simulink model "fcn"  (R2019a)
settings: Solver=VariableStepAuto  StartTime=0.0  StopTime=100  RelTol=1e-3
values from neighbouring files (symbols this model uses):
  x0 = [0;0;0;0]    [Script.m]
undefined symbols (not defined in the file or in its folder): params
settings Model: Creator=pc  LastModifiedBy=pc

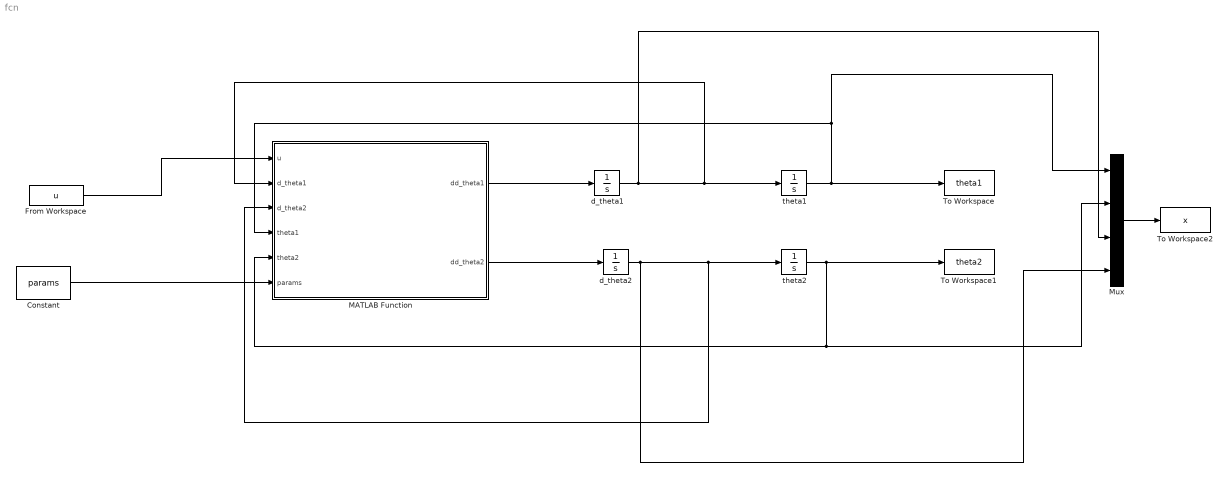
== system fcn ==
  Constant : Constant  Value=params  OutDataTypeStr=Bus: params_bus
  From Workspace : FromWorkspace  VariableName=u  SampleTime=0
  MATLAB Function : MATLAB Function  TreatAsAtomicUnit=on
  Mux : Mux
  To Workspace : ToWorkspace  VariableName=theta1  SaveFormat=Timeseries  SampleTime=-1
  To Workspace1 : ToWorkspace  VariableName=theta2  SaveFormat=Timeseries  SampleTime=-1
  To Workspace2 : ToWorkspace  VariableName=x  SaveFormat=Timeseries  SampleTime=-1
  d_theta1 : Integrator  InitialCondition=x0(2)
  d_theta2 : Integrator  InitialCondition=x0(4)
  theta1 : Integrator  InitialCondition=x0(1)
  theta2 : Integrator  InitialCondition=x0(3)
  wires:
  MATLAB Function/1(dd_theta1) -> d_theta1/1
  MATLAB Function/2(dd_theta2) -> d_theta2/1
  theta2/1 -> Mux/2, MATLAB Function/5(theta2), To Workspace1/1
  Constant/1 -> MATLAB Function/6(params)
  From Workspace/1 -> MATLAB Function/1(u)
  theta1/1 -> Mux/1, MATLAB Function/4(theta1), To Workspace/1
  d_theta1/1 -> Mux/3, MATLAB Function/2(d_theta1), theta1/1
  d_theta2/1 -> theta2/1, MATLAB Function/3(d_theta2), Mux/4
  Mux/1 -> To Workspace2/1

== matlab function fcn/MATLAB Function ==
  data: u input; dd_theta1 output; d_theta1 input; d_theta2 input; theta1 input; theta2 input; params input; dd_theta2 output
function [dd_theta1, dd_theta2] = fcn(u,d_theta1,d_theta2,theta1, theta2, params)

A = (-1)*d_theta2*d_theta2*sin(theta1 - theta2) - 2*(params.g/params.l)*sin(theta1) - params.zeta*d_theta1 + 1/(params.m*params.l*params.l)*u;
B = d_theta1*d_theta1*sin(theta1 - theta2) - (params.g/params.l)*sin(theta2) - params.zeta*d_theta2;
dd_theta1 = (B*cos(theta1-theta2)-A)/ ((-1)*cos(2*(theta1 - theta2)));
dd_theta2 = (2*B-A*cos(theta1 - theta2)) / (cos(2*(theta1 - theta2)));

end
